simulink model "aula20"  (R2021a)
settings: Solver=VariableStepAuto  StartTime=0.0  StopTime=3  MaxStep=0.05  RelTol=1e-3
settings Model: Creator=caue  LastModifiedBy=caue

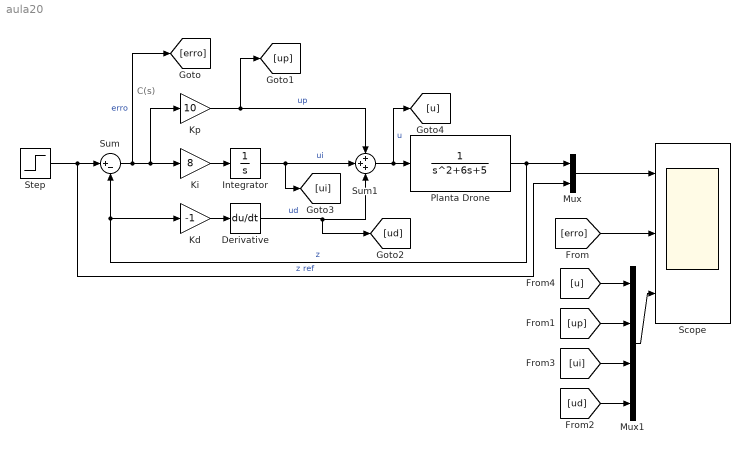
== system aula20 ==
  note: C(s)
  Derivative : Derivative
  Integrator : Integrator
  Kd : Gain  Gain=-1
  Ki : Gain  Gain=8
  Kp : Gain  Gain=10
  Mux : Mux  Inputs=2
  Mux1 : Mux
  Planta Drone : TransferFcn  Denominator=[1 6 5]
  Scope : Scope  NumInputPorts=3
  Step : Step  Time=0.1  SampleTime=0
  Sum : Sum  Inputs=|+-
  Sum1 : Sum  Inputs=+++
  wires:
  Step/1 -> Mux/2, Sum/1  "z ref"
  Sum/1 -> [erro], Ki/1, Kp/1  "erro"
  Ki/1 -> Integrator/1
  Kd/1 -> Derivative/1
  Integrator/1 -> Sum1/2, [ui]  "ui"
  Kp/1 -> [up], Sum1/1  "up"
  Derivative/1 -> Sum1/3, [ud]  "ud"
  Sum1/1 -> [u], Planta Drone/1  "u"
  Planta Drone/1 -> Mux/1, Kd/1, Sum/2  "z"
  Mux/1 -> Scope/1
  Mux1/1 -> Scope/3
  [erro] -> Scope/2
  [up] -> Mux1/2
  [ud] -> Mux1/4
  [ui] -> Mux1/3
  [u] -> Mux1/1
